simulink model "PIControlWithObserverR2"  (R2022a)
settings: Solver=VariableStepAuto  StartTime=0.0  StopTime=Tsim  FixedStep=dTMax  MaxStep=dTMax  RelTol=1e-3
values from neighbouring files (symbols this model uses):
  A = [A11 A12;A21 A22]    [VmPIWithObserverDriver_02Dec2022.m]    (also in observer_coeff.m)
  a1 = -1    [VmPIWithObserverDriver_02Dec2022.m]    (also in pi_controller_coeff.m = 0)
  a2 = 0    [VmPIWithObserverDriver_02Dec2022.m]
  Ao = [A11 A12;A21 A22]    [VmPIWithObserverDriver_02Dec2022.m]    (also in observer_coeff.m)
  B = [B11;B21]    [VmPIWithObserverDriver_02Dec2022.m]    (also in observer_coeff.m)
  b0 = Gcd.num{1}(1)    [VmPIWithObserverDriver_02Dec2022.m]    (also in pi_controller_coeff.m = 1)
  b1 = Gcd.num{1}(2)    [VmPIWithObserverDriver_02Dec2022.m]    (also in pi_controller_coeff.m = 0)
  b2 = 0    [VmPIWithObserverDriver_02Dec2022.m]
  Bo = [B11;B21]    [VmPIWithObserverDriver_02Dec2022.m]    (also in observer_coeff.m)
  C = [C11 C12;C21 C22;C31 C32]    [VmPIWithObserverDriver_02Dec2022.m]    (also in observer_coeff.m)
  Co = [C21 C22;C31 C32]    [VmPIWithObserverDriver_02Dec2022.m]    (also in observer_coeff.m)
  D = zeros(3,1)    [VmPIWithObserverDriver_02Dec2022.m]    (also in observer_coeff.m)
  L = placeO(Ao,Co,pDes)    [VmPIWithObserverDriver_02Dec2022.m]    (also in observer_coeff.m)
  N = 3    [VmPIWithObserverDriver_02Dec2022.m]
  Ts = 1/(MSPS*1e6)    (= 2e-07)    [VmPIWithObserverDriver_02Dec2022.m]
  VmDes = 0.05    [VmPIWithObserverDriver_02Dec2022.m]
  x0 = [0.1*VmDes 0]'    [VmPIWithObserverDriver_02Dec2022.m]
settings Model: Creator=seco6437  LastModifiedBy=koer2434
settings DebuggingCC: UnconnectedInputMsg=warning  UnconnectedOutputMsg=warning  UnconnectedLineMsg=warning
settings RTWCC: DLArmComputeVersion=19.05

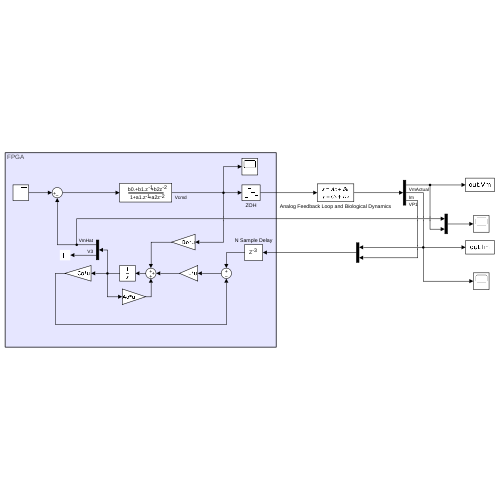
[thumbnail: Simulink's stored preview of the top-level diagram]
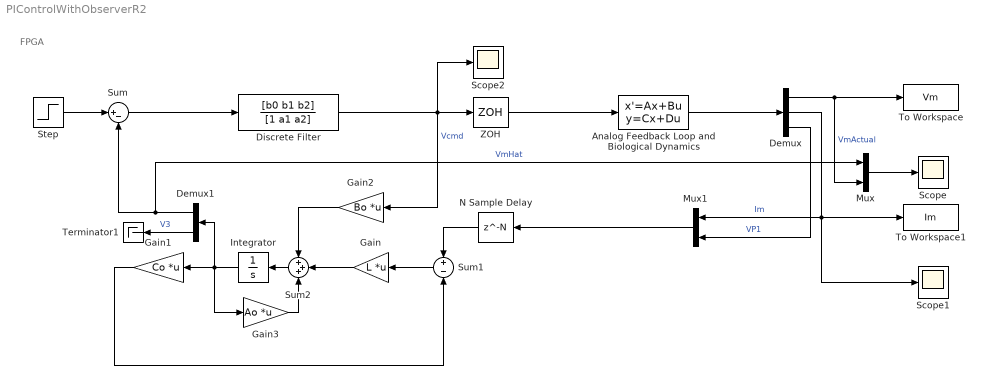
== system PIControlWithObserverR2 ==
  note: FPGA
  Analog Feedback Loop and Biological Dynamics : StateSpace  A=A  B=B  C=C  D=D  InitialCondition=x0
  Demux : Demux  Outputs=3
  Demux1 : Demux  Outputs=2
  Discrete Filter : DiscreteFilter  Numerator=[b0 b1 b2]  Denominator=[1 a1 a2]  SampleTime=Ts
  Gain : Gain  Gain=L  Multiplication=Matrix(K*u)
  Gain1 : Gain  Gain=Co  Multiplication=Matrix(K*u)
  Gain2 : Gain  Gain=Bo  Multiplication=Matrix(K*u)
  Gain3 : Gain  Gain=Ao  Multiplication=Matrix(K*u)
  Integrator : Integrator
  Mux : Mux  Inputs=2
  Mux1 : Mux  Inputs=2
  N Sample Delay : Delay  DelayLength=N  SampleTime=Ts
  Scope : Scope
  Scope1 : Scope
  Scope2 : Scope
  Step : Step  Time=0  After=VmDes  SampleTime=0
  Sum : Sum  Inputs=|+-
  Sum1 : Sum  Inputs=+|-
  Sum2 : Sum  Inputs=+++
  Terminator1 : Terminator
  To Workspace : ToWorkspace  VariableName=Vm  SaveFormat=Timeseries  SampleTime=-1
  To Workspace1 : ToWorkspace  VariableName=Im  SaveFormat=Timeseries  SampleTime=-1
  ZOH : ZeroOrderHold  SampleTime=Ts
  wires:
  Analog Feedback Loop and Biological Dynamics/1 -> Demux/1
  Step/1 -> Sum/1
  Discrete Filter/1 -> Scope2/1, ZOH/1, Gain2/1  "Vcmd"
  Sum1/1 -> Gain/1
  Integrator/1 -> Gain3/1, Demux1/1, Gain1/1
  Gain1/1 -> Sum1/2
  Sum2/1 -> Integrator/1
  Gain2/1 -> Sum2/1
  Gain3/1 -> Sum2/3
  Gain/1 -> Sum2/2
  Sum/1 -> Discrete Filter/1
  N Sample Delay/1 -> Sum1/1
  ZOH/1 -> Analog Feedback Loop and Biological Dynamics/1
  Mux/1 -> Scope/1
  Demux1/1 -> Mux/1, Sum/2  "VmHat"
  Demux1/2 -> Terminator1/1  "V3"
  Demux/1 -> Mux/2, To Workspace/1  "VmActual"
  Demux/2 -> Scope1/1, To Workspace1/1, Mux1/1  "Im"
  Mux1/1 -> N Sample Delay/1
  Demux/3 -> Mux1/2  "VP1"
